simulink model "open_buck_template"  (R2022a)
settings: Solver=ode45  StartTime=0.0  StopTime=0.01  MaxStep=0.1e-6  RelTol=1e-3  EnableMultiTasking=on
settings Model: Creator=Rieri  LastModifiedBy=emman
settings SolverCC: AlgebraicLoopSolver=TrustRegion
settings DataIOCC: LimitDataPoints=on  SaveFormat=Array  SignalLoggingSaveFormat=ModelDataLogs  ReturnWorkspaceOutputs=off
settings DebuggingCC: SaveWithParameterizedLinksMsg=none  UnderspecifiedInitializationDetection=Classic  MergeDetectMultiDrivingBlocksExec=none  SignalResolutionControl=TryResolveAllWithWarning  MultiTaskDSMMsg=warning  MultiTaskCondExecSysMsg=none  UnconnectedInputMsg=warning  UnconnectedOutputMsg=warning  UnconnectedLineMsg=warning  SFMachineParentedDataDiag=warning
settings HardwareCC: TargetUnknown=on
settings ModelReferenceCC: PropagateSignalLabelsOutOfModel=off
settings RTWCC: DLArmComputeVersion=19.05
settings GRTTargetCC: CombineOutputUpdateFcns=off  GRTInterface=on

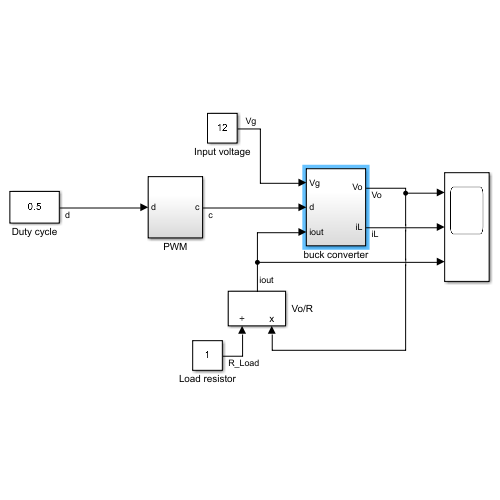
[thumbnail: Simulink's stored preview of the top-level diagram]
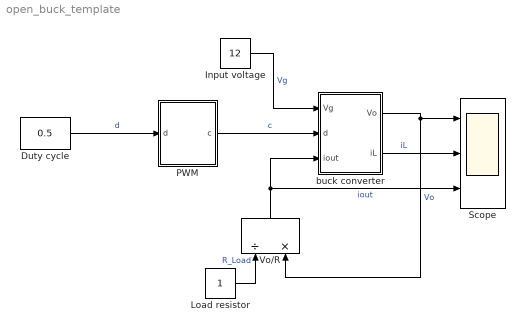
== system open_buck_template ==
  Duty cycle : Constant  Value=0.5
  Input voltage : Constant  Value=12
  Load resistor : Constant
  PWM : Subsystem
  Scope : Scope  NumInputPorts=3
  Vo/R : Product  Inputs=/*  SaturateOnIntegerOverflow=on
  buck converter : Subsystem
  wires:
  Input voltage/1 -> buck converter/1(Vg)  "Vg"
  buck converter/1(Vo) -> Scope/1, Vo/R/2  "Vo"
  buck converter/2(iL) -> Scope/2  "iL"
  Load resistor/1 -> Vo/R/1  "R_Load"
  Vo/R/1 -> Scope/3, buck converter/3(iout)  "iout"
  Duty cycle/1 -> PWM/1(d)  "d"
  PWM/1(c) -> buck converter/2(d)  "c"

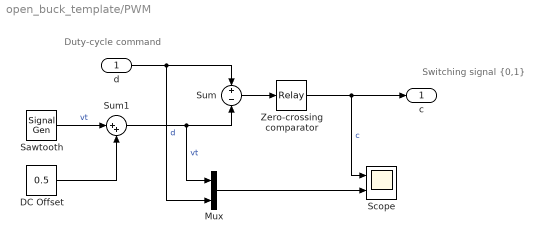
== system open_buck_template/PWM ==
  note: Duty-cycle
      | command
  note: Switching signal {0,1}
  d : Inport
  DC Offset : Constant  Value=0.5
  Mux : Mux  Inputs=2
  Sawtooth : SignalGenerator  WaveForm=sawtooth  Amplitude=-0.5  Frequency=100000
  Scope : Scope  NumInputPorts=2
  Sum : Sum  Inputs=+|-  SaturateOnIntegerOverflow=on
  Sum1 : Sum  Inputs=|++
  Zero-crossing comparator : Relay
  c : Outport
  wires:
  Sum1/1 -> Mux/1, Sum/2  "vt"
  d/1 -> Mux/2, Sum/1  "d"
  Zero-crossing comparator/1 -> c/1, Scope/1  "c"
  Sum/1 -> Zero-crossing comparator/1
  Mux/1 -> Scope/2
  Sawtooth/1 -> Sum1/1  "vt"
  DC Offset/1 -> Sum1/2

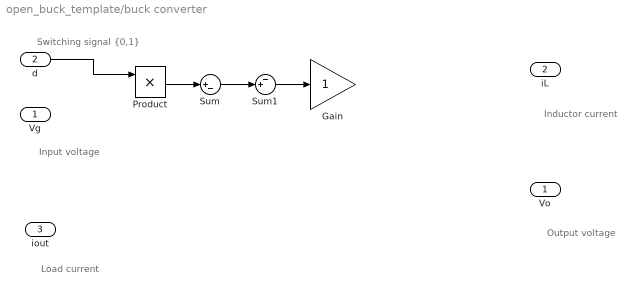
== system open_buck_template/buck converter ==
  note: Load current
  note: Input voltage
  note: Inductor current
  note: Output voltage
  note: Switching signal {0,1}
  Vg : Inport
  d : Inport  Port=2
  iout : Inport  Port=3
  Gain : Gain
  Product : Product
  Sum : Sum  Inputs=|+-
  Sum1 : Sum  Inputs=-+|
  Vo : Outport
  iL : Outport  Port=2
  wires:
  d/1 -> Product/1
  Product/1 -> Sum/1
  Sum/1 -> Sum1/2
  Sum1/1 -> Gain/1
